simulink model "SX_Hand"  (R2014a)
settings: Solver=ode3  StartTime=0.0  StopTime=40  RelTol=1e-3
settings Model: Creator=Tonno  LastModifiedBy=Tonno
settings OptimizationCC: OptimizeModelRefInitCode=on  LifeSpan=1
settings RTWCC: SystemTargetFile=ert.tlc  GenCodeOnly=on  TemplateMakefile=ert_default_tmf  Description=Embedded Coder  ProcessScript=ert_make_rtw_hook
settings CodeAppCC: IgnoreCustomStorageClasses=off  CustomSymbolStrType=$N$R$M_SymType  InternalIdentifier=Classic
settings ERTTargetCC: ParMdlRefBuildCompliant=on  CompOptLevelCompliant=on  ConcurrentExecutionCompliant=on  ERTFirstTimeCompliant=on  SupportAbsoluteTime=off  MultiInstanceERTCode=on  CodeInterfacePackaging=Reusable function  SupportNonFinite=off  SupportComplex=off  ModelStepFunctionPrototypeControlCompliant=on  CPPClassGenCompliant=on  InlinedParameterPlacement=Hierarchical  RootIOFormat=Structure reference  ERTCustomFileTemplate=example_file_process.tlc

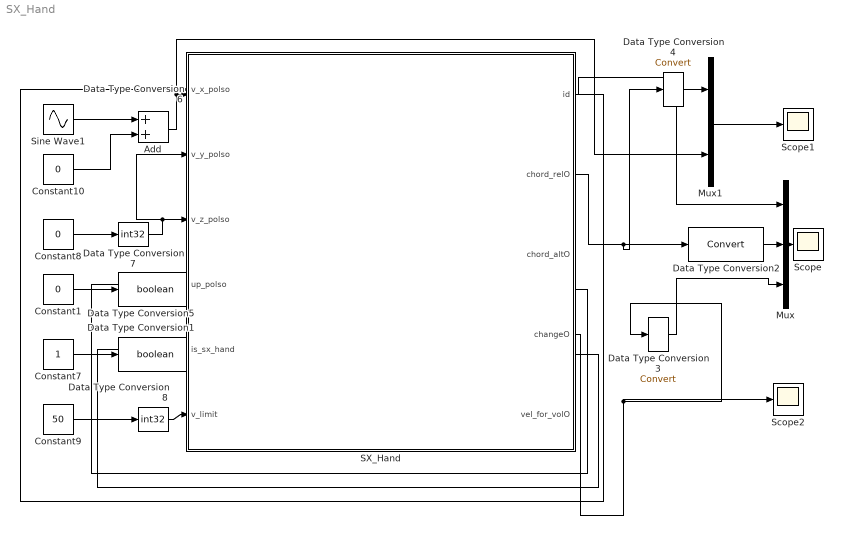
== system SX_Hand ==
  Add : Sum
  Constant1 : Constant  Value=0
  Constant10 : Constant  Value=0
  Constant7 : Constant
  Constant8 : Constant  Value=0
  Constant9 : Constant  Value=50
  Data Type Conversion1 : DataTypeConversion  OutDataTypeStr=boolean
  Data Type Conversion2 : DataTypeConversion
  Data Type Conversion3 : DataTypeConversion
  Data Type Conversion4 : DataTypeConversion
  Data Type Conversion5 : DataTypeConversion  OutDataTypeStr=boolean
  Data Type Conversion6 : DataTypeConversion  OutDataTypeStr=int32
  Data Type Conversion7 : DataTypeConversion  OutDataTypeStr=int32
  Data Type Conversion8 : DataTypeConversion  OutDataTypeStr=int32
  Mux : Mux  Inputs=3
  Mux1 : Mux  Inputs=2
  SX_Hand : Stateflow chart  TreatAsAtomicUnit=on
  Scope : Scope
      settings: YMin=0  YMax=17000
  Scope1 : Scope
      settings: TimeRange=20  YMin=-6  YMax=6
  Scope2 : Scope
      settings: YMin=0  YMax=17000  SaveName=ScopeData2
  Sine Wave1 : Sin  Amplitude=100  Frequency=0.5  SampleTime=0
  wires:
  SX_Hand/2(chord_relO) -> Data Type Conversion4/1, Data Type Conversion2/1
  SX_Hand/1(id) -> Mux/1
  Mux/1 -> Scope/1
  Constant7/1 -> Data Type Conversion1/1
  Data Type Conversion1/1 -> SX_Hand/5(is_sx_hand)
  Data Type Conversion2/1 -> Mux/2
  Data Type Conversion3/1 -> Mux/3
  Mux1/1 -> Scope1/1
  Data Type Conversion4/1 -> Mux1/1
  Sine Wave1/1 -> Add/1
  Constant10/1 -> Add/2
  Add/1 -> Data Type Conversion6/1, Mux1/2
  Constant1/1 -> Data Type Conversion5/1
  Data Type Conversion5/1 -> SX_Hand/4(up_polso)
  Constant9/1 -> Data Type Conversion8/1
  Constant8/1 -> Data Type Conversion7/1
  Data Type Conversion6/1 -> SX_Hand/1(v_x_polso)
  Data Type Conversion7/1 -> SX_Hand/2(v_y_polso), SX_Hand/3(v_z_polso)
  Data Type Conversion8/1 -> SX_Hand/6(v_limit)
  SX_Hand/4(changeO) -> Scope2/1, Data Type Conversion3/1

== stateflow chart SX_Hand/SX_Hand ==
  state Chord_change_control [parallel]
    during: changeO = false;
    settings: executionOrder=1
    state playing_mode
      state filter_state
        entry: changeO=true;
        entry: id=id+1;
        entry: chord_relO=chord_relL;
        entry: vel_for_volO=vel_for_volL;
      state wait_for_change
      filter_state -> wait_for_change : [not(up_polso) && (v_x_polso > (-v_limit)) && (v_x_polso < v_limit) && (v_y_polso > (-v_limit)) && (v_y_polso < v_limit) && (v_z_polso > (-v_limit)) &&(v_z_polso < v_limit)]
      wait_for_change -> filter_state [order 2] : [v_x_polso < (-v_limit)] /{chord_relL= uint8(3);vel_for_volL=abs(v_x_polso);}
      wait_for_change -> filter_state [order 1] : [v_x_polso > v_limit] /{chord_relL= uint8(1);vel_for_volL=abs(v_x_polso);}
      wait_for_change -> filter_state [order 6] : [v_y_polso < (-v_limit)] /{chord_relL= uint8(6); vel_for_volL=abs(v_y_polso);}
      wait_for_change -> filter_state [order 7] : [up_polso]/{chord_relL= uint8(7); vel_for_volL= int32(500);}
      wait_for_change -> filter_state [order 4] : [v_z_polso < (-v_limit)] /{chord_relL= uint8(2);vel_for_volL=abs(v_z_polso);}
      wait_for_change -> filter_state [order 5] : [v_y_polso > v_limit] /{chord_relL= uint8(5);vel_for_volL=abs(v_y_polso);}
      wait_for_change -> filter_state [order 3] : [v_z_polso > v_limit]/{chord_relL = uint8(4);vel_for_volL=abs(v_z_polso);}
    state wait_hand
      entry: id=id+1;
      entry: changeO=true;
      entry: chord_relO = uint8(0);
      entry: chord_relL = uint8(0);
      entry: vel_for_volL = int32(0);
      entry: vel_for_volO = int32(0);
    wait_hand -> wait_for_change : [is_sx_hand]
    (default) -> wait_hand : /{id= uint16(0);}
    playing_mode -> wait_hand : [not(is_sx_hand)]
  state Alterations_control [parallel]
    settings: executionOrder=2
    state no_alt
      en: chord_altO= uint8(0);
    (default) -> no_alt
  data: id output uint16; chord_relO output uint8; chord_altO output uint8; v_x_polso input int32; v_y_polso input int32; v_z_polso input int32; up_polso input boolean; changeO output boolean; is_sx_hand input boolean; v_limit input int32; chord_relL local uint8; vel_for_volO output int32; vel_for_volL local int32
  events: tick local RISING_EDGE_EVENT
